simulink model "filecuaho"  (R2016b)
settings: Solver=VariableStepAuto  StartTime=0.0  StopTime=10.0  RelTol=1e-3
undefined symbols (not defined in the file): KACC_ACCT_CLR_NIDL_INIT, KACC_ACCUT_STATE_A, KACC_ACCUT_STATE_B, KACC_ACCUT_SW, KACC_ACTQSW, KACC_CLD, KACC_CLD_REQ_HYS, KACC_CLD_REQ_SW, KACC_COLPD, KACC_COMP_INRT, KACC_COMPTYPE_FIXED, KACC_COMPTYPE_VAR, KACC_CTTM_ACE, KACC_CTTM_ACON, KACC_CTTM_CRK, KACC_CTTM_FAN, KACC_CTTM_GRD, KACC_CTTM_IRS, KACC_CTTM_NAC, KACC_DIFFEVATEMPMAX, KACC_DIFFEVATEMPMIN, KACC_EVAT_ELSE, KACC_EVAT_ELSE_SW, KACC_EVATMPCUT_SW, KACC_EVATUPL_ELSE, KACC_EVATUPL_ELSE_SW, KACC_FANREQ_SW, KACC_FORCEDACON, KACC_HCAPS, KACC_HCAPS_HYS, KACC_HCCTTM, KACC_HCGRA, KACC_HCGRA_HYS, KACC_HCRGR, KACC_HCVS1, KACC_HCVS1_HYS, KACC_HCVS2, KACC_HCVS2_HYS, KACC_HEATUP_CE, KACC_HEATUP_CE_HYS, KACC_HEATUP_DRV2IDL, KACC_HEATUP_IDL2DRV, KACC_HEATUP_NE, KACC_HEATUP_NE_HYS, KACC_HIPS_ACOF, KACC_HIPS_ACON, KACC_LOPS_ACOF, KACC_LOPS_ACON, KACC_LYR3TR_ACHLD, KACC_NEW_RPM, KACC_OFDL_SW, KACC_OFDL_VCV, KACC_ONDL_SW, KACC_RECCP, KACC_RECCP_HYS, KACC_RECDLY, KACC_RECVS, KACC_S1_THWMAX, KACC_S1TM_THWULMT, KACC_SHLT_2CYL ... (+137)
libraries: lib2011b x727, SUBSYSTEM_LIB_CNV x30, SUBSYSTEM_LIB_ESC x2, SUBSYSTEM_LIB_AUX x1
(part 4 of 5)

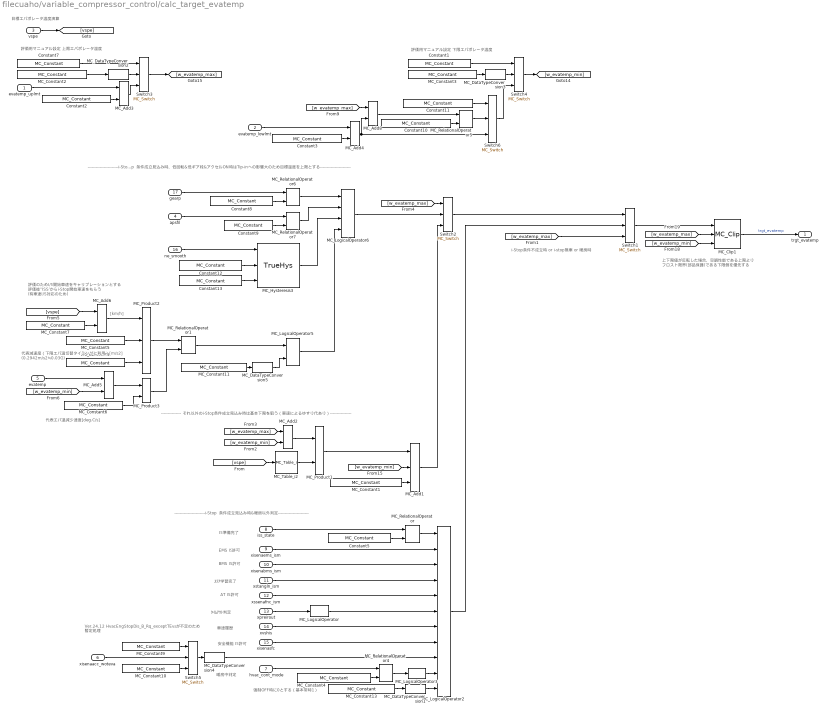
== system filecuaho/variable_compressor_control/calc_target_evatemp ==
  note: 評価用マニュアル設定 上限エバポレータ温度
  note: 評価用マニュアル設定 下限エバポレータ温度
  note: 上下限値が反転した場合、空調性能である上限より
      | フロスト限界(部品保護)である下限側を優先する
  note: 目標エバポレータ温度演算
  note: i-Stop条件不成立時 or i-stop無車 or 暖房時
  note: ---------------それ以外のi-Stop条件成立見込み時は基本下限を狙う（車速によるゆすり代あり）----------------
  note: -----------------------i-Stop条件成立見込み時、低回転&低ギア段&アクセルON時はTip-inへの影響大のため目標温度を上限とする-----------------------
  note: 代表減速度（下限エバ温切替タイミングに利用）[m/s2]
      | (0.2942m/s2≒0.03G)
  note: 代表エバ温減少速度[deg.C/s]
  note: 評価のためI/S開始車速をキャリブレーションとする
      | 評価後"ISS"からi-Stop開始車速をもらう
      | (有車速I/S対応のため)
  note: [km/h]
  note: Ver.24.12
      | HvacEngStopDis_B_Rq_exceptTEvaが不定のため
      | 暫定処理
  note: EMS IS許可
  note: BMS IS許可
  note: ｽﾃｱ学習完了
  note: AT IS許可
  note: ﾀｲﾑｱｳﾄ判定
  note: 車速履歴
  note: 安全機能 IS許可
  note: IS準備完了
  note: -----------------------i-Stop条件成立見込み時&暖房以外判定-----------------------
  note: 暖房中判定
  note: 強制OFF時に0とする（基本常時1）
  evatemp_uplmt : Inport
  evatemp_lowlmt : Inport  Port=2
  vspe : Inport  Port=3
  apsfil : Inport  Port=4
  evatemp : Inport  Port=5
  xisenaacc_woteva : Inport  Port=6
  hvac_cont_mode : Inport  Port=7
  iss_state : Inport  Port=8
  xisenaems_ism : Inport  Port=9
  xisenabms_ism : Inport  Port=10
  xstangln_ism : Inport  Port=11
  xssenafnc_ism : Inport  Port=12
  xpreirout : Inport  Port=13
  xvshis : Inport  Port=14
  xisenasfc : Inport  Port=15
  ne_smooth : Inport  Port=16
  gearp : Inport  Port=17
  Constant1 : lib2011b/Simulink Original/Sources/MC_Constant  Value=KACC_VCD_ETLO_MN  datatype=Inherit: Inherit from 'Constant value'  SampleTime=inf  FramePeriod=inf  OutMin=[]  OutMax=[]  OutDataTypeStr=Inherit: Inherit from 'Constant value'
  Constant10 : lib2011b/Simulink Original/Sources/MC_Constant  Value=KACC_VCD_EVA_DIFTEMP  datatype=Inherit: Inherit from 'Constant value'  SampleTime=inf  FramePeriod=inf  OutMin=[]  OutMax=[]  OutDataTypeStr=Inherit: Inherit from 'Constant value'
  Constant11 : lib2011b/Simulink Original/Sources/MC_Constant  Value=KACC_VCD_ETLO_TEMP  datatype=Inherit: Inherit from 'Constant value'  SampleTime=inf  FramePeriod=inf  OutMin=[]  OutMax=[]  OutDataTypeStr=Inherit: Inherit from 'Constant value'
  Constant12 : lib2011b/Simulink Original/Sources/MC_Constant  Value=KACC_VCD_NE  datatype=Inherit: Inherit from 'Constant value'  SampleTime=inf  FramePeriod=inf  OutMin=[]  OutMax=[]  OutDataTypeStr=Inherit: Inherit from 'Constant value'
  Constant13 : lib2011b/Simulink Original/Sources/MC_Constant  Value=KACC_VCD_NE_HYS  datatype=Inherit: Inherit from 'Constant value'  SampleTime=inf  FramePeriod=inf  OutMin=[]  OutMax=[]  OutDataTypeStr=Inherit: Inherit from 'Constant value'
  Constant2 : lib2011b/Simulink Original/Sources/MC_Constant  Value=KACC_VCD_ETHI_OFST  datatype=Inherit: Inherit from 'Constant value'  SampleTime=inf  FramePeriod=inf  OutMin=[]  OutMax=[]  OutDataTypeStr=Inherit: Inherit from 'Constant value'
  Constant3 : lib2011b/Simulink Original/Sources/MC_Constant  Value=KACC_VCD_ETLO_OFST  datatype=Inherit: Inherit from 'Constant value'  SampleTime=inf  FramePeriod=inf  OutMin=[]  OutMax=[]  OutDataTypeStr=Inherit: Inherit from 'Constant value'
  Constant5 : lib2011b/Simulink Original/Sources/MC_Constant  Value=KACC_VCD_ISNOTRDY  datatype=Inherit: Inherit from 'Constant value'  SampleTime=inf  FramePeriod=inf  OutMin=[]  OutMax=[]  OutDataTypeStr=Inherit: Inherit from 'Constant value'
  Constant7 : lib2011b/Simulink Original/Sources/MC_Constant  Value=KACC_VCD_ETHI_MN  datatype=Inherit: Inherit from 'Constant value'  SampleTime=inf  FramePeriod=inf  OutMin=[]  OutMax=[]  OutDataTypeStr=Inherit: Inherit from 'Constant value'
  Constant8 : lib2011b/Simulink Original/Sources/MC_Constant  Value=KACC_VCD_GEARP  datatype=Inherit: Inherit from 'Constant value'  SampleTime=inf  FramePeriod=inf  OutMin=[]  OutMax=[]  OutDataTypeStr=Inherit: Inherit from 'Constant value'
  Constant9 : lib2011b/Simulink Original/Sources/MC_Constant  Value=KACC_VCD_APS  datatype=Inherit: Inherit from 'Constant value'  SampleTime=inf  FramePeriod=inf  OutMin=[]  OutMax=[]  OutDataTypeStr=Inherit: Inherit from 'Constant value'
  MC_Add1 : lib2011b/Simulink Original/Math Operations/MC_Add  Inputs=+++  CollapseDim=1  SampleTime=-1  InputSameDT=on  OutMin=[]  OutMax=[]  OutDataTypeStr=single
  MC_Add{2,5..6,8} (4 alike) : lib2011b/Simulink Original/Math Operations/MC_Add  Inputs=+-  CollapseDim=1  SampleTime=-1  InputSameDT=on  OutMin=[]  OutMax=[]  OutDataTypeStr=single
  MC_Add3 : lib2011b/Simulink Original/Math Operations/MC_Add  Inputs=++  CollapseDim=1  SampleTime=-1  InputSameDT=on  OutMin=[]  OutMax=[]  OutDataTypeStr=single
  MC_Add4 : lib2011b/Simulink Original/Math Operations/MC_Add  Inputs=++  CollapseDim=1  SampleTime=-1  InputSameDT=on  OutMin=[]  OutMax=[]  OutDataTypeStr=single
  MC_Clip1 : lib2011b/Mazda Library/Other/MC_Clip
  MC_Constant1 : lib2011b/Simulink Original/Sources/MC_Constant  Value=KACC_VCD_TET_OFFSET  datatype=Inherit: Inherit from 'Constant value'  SampleTime=inf  FramePeriod=inf  OutMin=[]  OutMax=[]  OutDataTypeStr=Inherit: Inherit from 'Constant value'
  MC_Constant10 : lib2011b/Simulink Original/Sources/MC_Constant  Value=KACC_VCD_ISOFF  datatype=Inherit: Inherit from 'Constant value'  SampleTime=inf  FramePeriod=inf  OutMin=[]  OutMax=[]  OutDataTypeStr=Inherit: Inherit from 'Constant value'
  MC_Constant11 : lib2011b/Simulink Original/Sources/MC_Constant  Value=KACC_VCD_EVASP_SW  datatype=Inherit: Inherit from 'Constant value'  SampleTime=inf  FramePeriod=inf  OutMin=[]  OutMax=[]  OutDataTypeStr=Inherit: Inherit from 'Constant value'
  MC_Constant13 : lib2011b/Simulink Original/Sources/MC_Constant  Value=KACC_VCD_FORCEDOFF  datatype=Inherit: Inherit from 'Constant value'  SampleTime=inf  FramePeriod=inf  OutMin=[]  OutMax=[]  OutDataTypeStr=Inherit: Inherit from 'Constant value'
  MC_Constant2 : lib2011b/Simulink Original/Sources/MC_Constant  Value=KACC_VCD_ETHI_MNSW  datatype=Inherit: Inherit from 'Constant value'  SampleTime=inf  FramePeriod=inf  OutMin=[]  OutMax=[]  OutDataTypeStr=Inherit: Inherit from 'Constant value'
  MC_Constant3 : lib2011b/Simulink Original/Sources/MC_Constant  Value=KACC_VCD_ETLO_MNSW  datatype=Inherit: Inherit from 'Constant value'  SampleTime=inf  FramePeriod=inf  OutMin=[]  OutMax=[]  OutDataTypeStr=Inherit: Inherit from 'Constant value'
  MC_Constant4 : lib2011b/Simulink Original/Sources/MC_Constant  Value=KACC_VCD_HEATSTATE2  datatype=Inherit: Inherit from 'Constant value'  SampleTime=inf  FramePeriod=inf  OutMin=[]  OutMax=[]  OutDataTypeStr=Inherit: Inherit from 'Constant value'
  MC_Constant5 : lib2011b/Simulink Original/Sources/MC_Constant  Value=KACC_VCD_DISACC  datatype=Inherit: Inherit from 'Constant value'  SampleTime=inf  FramePeriod=inf  OutMin=[]  OutMax=[]  OutDataTypeStr=Inherit: Inherit from 'Constant value'
  MC_Constant6 : lib2011b/Simulink Original/Sources/MC_Constant  Value=KACC_VCD_DISET  datatype=Inherit: Inherit from 'Constant value'  SampleTime=inf  FramePeriod=inf  OutMin=[]  OutMax=[]  OutDataTypeStr=Inherit: Inherit from 'Constant value'
  MC_Constant7 : lib2011b/Simulink Original/Sources/MC_Constant  Value=KACC_VCD_ISSPD  datatype=Inherit: Inherit from 'Constant value'  SampleTime=inf  FramePeriod=inf  OutMin=[]  OutMax=[]  OutDataTypeStr=Inherit: Inherit from 'Constant value'
  MC_Constant8 : lib2011b/Simulink Original/Sources/MC_Constant  Value=3.6  datatype=single  SampleTime=inf  FramePeriod=inf  OutMin=[]  OutMax=[]  OutDataTypeStr=single
  MC_Constant9 : lib2011b/Simulink Original/Sources/MC_Constant  Value=KACC_VCD_ISON  datatype=Inherit: Inherit from 'Constant value'  SampleTime=inf  FramePeriod=inf  OutMin=[]  OutMax=[]  OutDataTypeStr=Inherit: Inherit from 'Constant value'
  MC_DataTypeConversion{1..5} (5 alike) : lib2011b/Simulink Original/Signal Attributes/MC_DataTypeConversion  OutMin=[]  OutMax=[]  OutDataTypeStr=boolean  Signaltype=boolean  ConvertRealWorld=Real World Value (RWV)  RndMeth=Zero  SampleTime=-1
  MC_Hysteresis3 : SUBSYSTEM_LIB_CNV/TrueHys
      settings: AttributesFormatString=True
  MC_LogicalOperator : lib2011b/Simulink Original/Logic and Bit Operations/MC_LogicalOperator  SelectedOperator=NOT  Inputs=2  SampleTime=-1  AllPortsSameDT=off  OutDataTypeStr=boolean
  MC_LogicalOperator2 : lib2011b/Simulink Original/Logic and Bit Operations/MC_LogicalOperator  SelectedOperator=AND  Inputs=11  SampleTime=-1  AllPortsSameDT=off  OutDataTypeStr=boolean
  MC_LogicalOperator3 : lib2011b/Simulink Original/Logic and Bit Operations/MC_LogicalOperator  SelectedOperator=NOT  Inputs=2  SampleTime=-1  AllPortsSameDT=off  OutDataTypeStr=boolean
  MC_LogicalOperator5 : lib2011b/Simulink Original/Logic and Bit Operations/MC_LogicalOperator  SelectedOperator=OR  Inputs=2  SampleTime=-1  AllPortsSameDT=off  OutDataTypeStr=boolean
  MC_LogicalOperator6 : lib2011b/Simulink Original/Logic and Bit Operations/MC_LogicalOperator  SelectedOperator=AND  Inputs=4  SampleTime=-1  AllPortsSameDT=off  OutDataTypeStr=boolean
  MC_Product1 : lib2011b/Simulink Original/Math Operations/MC_Product  Inputs=**  Multiplication=Element-wise(.*)  CollapseDim=1  SampleTime=-1  InputSameDT=on  OutMin=[]  OutMax=[]  OutDataTypeStr=single  RndMeth=Zero
  MC_Product2 : lib2011b/Simulink Original/Math Operations/MC_Product  Inputs=*//  Multiplication=Element-wise(.*)  CollapseDim=1  SampleTime=-1  InputSameDT=on  OutMin=[]  OutMax=[]  OutDataTypeStr=single  RndMeth=Zero
  MC_Product3 : lib2011b/Simulink Original/Math Operations/MC_Product  Inputs=*/  Multiplication=Element-wise(.*)  CollapseDim=1  SampleTime=-1  InputSameDT=on  OutMin=[]  OutMax=[]  OutDataTypeStr=single  RndMeth=Zero
  MC_RelationalOperator : lib2011b/Simulink Original/Logic and Bit Operations/MC_RelationalOperator  Operator=~=  SampleTime=-1  InputSameDT=on  OutDataTypeStr=boolean
  MC_RelationalOperator1 : lib2011b/Simulink Original/Logic and Bit Operations/MC_RelationalOperator  Operator=>  SampleTime=-1  InputSameDT=on  OutDataTypeStr=boolean
  MC_RelationalOperator4 : lib2011b/Simulink Original/Logic and Bit Operations/MC_RelationalOperator  Operator===  SampleTime=-1  InputSameDT=on  OutDataTypeStr=boolean
  MC_RelationalOperator5 : lib2011b/Simulink Original/Logic and Bit Operations/MC_RelationalOperator  Operator=>=  SampleTime=-1  InputSameDT=on  OutDataTypeStr=boolean
  MC_RelationalOperator6 : lib2011b/Simulink Original/Logic and Bit Operations/MC_RelationalOperator  Operator=>=  SampleTime=-1  InputSameDT=on  OutDataTypeStr=boolean
  MC_RelationalOperator7 : lib2011b/Simulink Original/Logic and Bit Operations/MC_RelationalOperator  Operator=>  SampleTime=-1  InputSameDT=on  OutDataTypeStr=boolean
  MC_Table_i2 : lib2011b/Simulink Original/Lookup Tables/MC_Table_i  Label=TACC_VCD_TTEMP_VSP  InputValues=TACC_VCD_TTEMP_VSP_X  calsw_x=on  OutputValues=TACC_VCD_TTEMP_VSP_Y  LsbValue=LSB_TACC_VCD_TTEMP_VSP_Y  OffsetValue=OFFSET_TACC_VCD_TTEMP_VSP_Y
      settings: AttributesFormatString=%<Label>\nX-axis %<calsw_x>
  Switch{1..6} (6 alike) : lib2011b/Simulink Original/Signal Routing/MC_Switch  Criteria=u2 ~= 0  Threshold=0  SampleTime=-1  InputSameDT=on  OutMin=[]  OutMax=[]  AllowDiffInputSizes=off
  trgt_evatemp : Outport
  wires:
  [vspe] -> MC_Table_i2/1
  MC_Product1/1 -> MC_Add1/1
  MC_Constant1/1 -> MC_Add1/3
  MC_Add2/1 -> MC_Product1/1
  MC_Table_i2/1 -> MC_Product1/2
  MC_DataTypeConversion2/1 -> Switch3/2
  MC_Constant2/1 -> MC_DataTypeConversion2/1
  Constant7/1 -> Switch3/1
  MC_DataTypeConversion3/1 -> Switch4/2
  MC_Constant3/1 -> MC_DataTypeConversion3/1
  Constant1/1 -> Switch4/1
  Switch3/1 -> [w_evatemp_max]
  [w_evatemp_max] -> MC_Clip1/2
  [w_evatemp_min] -> MC_Clip1/3
  [w_evatemp_min] -> MC_Add1/2
  MC_Clip1/1 -> trgt_evatemp/1  "trgt_evatemp"
  Switch1/1 -> MC_Clip1/1
  [w_evatemp_max] -> MC_Add2/1
  [w_evatemp_min] -> MC_Add2/2
  Constant2/1 -> MC_Add3/2
  MC_Add3/1 -> Switch3/3
  Constant3/1 -> MC_Add4/2
  evatemp_lowlmt/1 -> MC_Add4/1
  vspe/1 -> [vspe]
  MC_Constant5/1 -> MC_Product2/2
  MC_Product2/1 -> MC_RelationalOperator1/1
  [w_evatemp_min] -> MC_Add5/2
  evatemp/1 -> MC_Add5/1
  MC_Constant6/1 -> MC_Product3/2
  MC_Product3/1 -> MC_RelationalOperator1/2
  MC_Add5/1 -> MC_Product3/1
  MC_Constant7/1 -> MC_Add6/2
  MC_Add6/1 -> MC_Product2/1
  [vspe] -> MC_Add6/1
  MC_Constant8/1 -> MC_Product2/3
  iss_state/1 -> MC_RelationalOperator/1
  Constant5/1 -> MC_RelationalOperator/2
  xpreirout/1 -> MC_LogicalOperator/1
  MC_Constant9/1 -> Switch5/1
  MC_Constant10/1 -> Switch5/3
  xisenaacc_woteva/1 -> Switch5/2
  Switch5/1 -> MC_DataTypeConversion4/1
  hvac_cont_mode/1 -> MC_RelationalOperator4/1
  MC_Constant4/1 -> MC_RelationalOperator4/2
  MC_Constant13/1 -> MC_DataTypeConversion1/1
  MC_RelationalOperator4/1 -> MC_LogicalOperator3/1
  MC_RelationalOperator/1 -> MC_LogicalOperator2/1
  xisenaems_ism/1 -> MC_LogicalOperator2/2
  xisenabms_ism/1 -> MC_LogicalOperator2/3
  xstangln_ism/1 -> MC_LogicalOperator2/4
  xssenafnc_ism/1 -> MC_LogicalOperator2/5
  MC_LogicalOperator/1 -> MC_LogicalOperator2/6
  xvshis/1 -> MC_LogicalOperator2/7
  xisenasfc/1 -> MC_LogicalOperator2/8
  MC_DataTypeConversion4/1 -> MC_LogicalOperator2/9
  MC_LogicalOperator3/1 -> MC_LogicalOperator2/10
  MC_DataTypeConversion1/1 -> MC_LogicalOperator2/11
  Switch2/1 -> Switch1/1
  MC_LogicalOperator2/1 -> Switch1/2
  [w_evatemp_max] -> Switch1/3
  MC_Constant11/1 -> MC_DataTypeConversion5/1
  MC_RelationalOperator1/1 -> MC_LogicalOperator5/1
  MC_DataTypeConversion5/1 -> MC_LogicalOperator5/2
  evatemp_uplmt/1 -> MC_Add3/1
  [w_evatemp_max] -> MC_Add8/1
  MC_Add8/1 -> MC_RelationalOperator5/1
  Constant10/1 -> MC_RelationalOperator5/2
  MC_Add4/1 -> MC_Add8/2, Switch6/3
  Constant11/1 -> Switch6/1
  MC_RelationalOperator5/1 -> Switch6/2
  Switch6/1 -> Switch4/3
  Switch4/1 -> [w_evatemp_min]
  gearp/1 -> MC_RelationalOperator6/1
  Constant8/1 -> MC_RelationalOperator6/2
  Constant9/1 -> MC_RelationalOperator7/2
  MC_RelationalOperator6/1 -> MC_LogicalOperator6/1
  MC_RelationalOperator7/1 -> MC_LogicalOperator6/2
  MC_LogicalOperator5/1 -> MC_LogicalOperator6/4
  apsfil/1 -> MC_RelationalOperator7/1
  MC_LogicalOperator6/1 -> Switch2/2
  [w_evatemp_max] -> Switch2/1
  MC_Add1/1 -> Switch2/3
  ne_smooth/1 -> MC_Hysteresis3/1
  Constant12/1 -> MC_Hysteresis3/2
  Constant13/1 -> MC_Hysteresis3/3
  MC_Hysteresis3/1 -> MC_LogicalOperator6/3

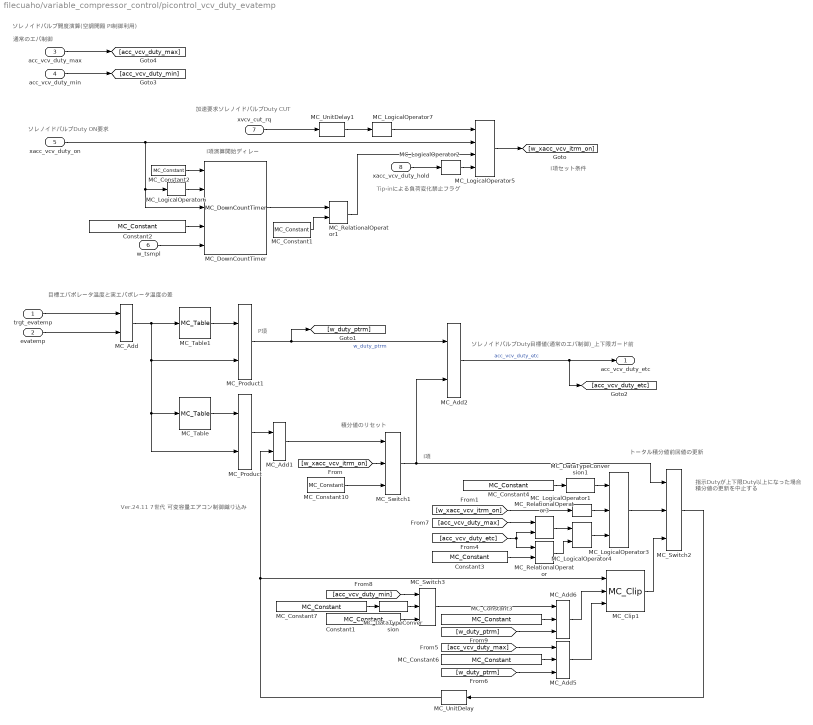
== system filecuaho/variable_compressor_control/picontrol_vcv_duty_evatemp ==
  note: 積分値のリセット
  note: 目標エバポレータ温度と実エバポレータ温度の差
  note: I項
  note: P項
  note: トータル積分値前回値の更新
  note: 通常のエバ制御
  note: ソレノイドバルブ開度演算(空調開殿 PI制御利用)
  note: 指示Dutyが上下限Duty以上になった場合
      | 積分値の更新を中止する
  note: ソレノイドバルブDuty目標値(通常のエバ制御)_上下限ガード前
  note: ソレノイドバルブDuty ON要求
  note: Ver.24.11
      | 7世代 可変容量エアコン制御織り込み
  note: I項セット条件
  note: I項演算開始ディレー
  note: 加速要求ソレノイドバルブDuty CUT
  note: Tip-inによる負荷変化禁止フラグ
  trgt_evatemp : Inport
  evatemp : Inport  Port=2
  acc_vcv_duty_max : Inport  Port=3
  acc_vcv_duty_min : Inport  Port=4
  xacc_vcv_duty_on : Inport  Port=5
  w_tsmpl : Inport  Port=6
  xvcv_cut_rq : Inport  Port=7
  xacc_vcv_duty_hold : Inport  Port=8
  Constant1 : lib2011b/Simulink Original/Sources/MC_Constant  Value=KACC_VCD_INIT  datatype=Inherit: Inherit from 'Constant value'  SampleTime=inf  FramePeriod=inf  OutMin=[]  OutMax=[]  OutDataTypeStr=Inherit: Inherit from 'Constant value'
  Constant2 : lib2011b/Simulink Original/Sources/MC_Constant  Value=KACC_VCD_ITSET_DLY  datatype=Inherit: Inherit from 'Constant value'  SampleTime=inf  FramePeriod=inf  OutMin=[]  OutMax=[]  OutDataTypeStr=Inherit: Inherit from 'Constant value'
  Constant3 : lib2011b/Simulink Original/Sources/MC_Constant  Value=KACC_VCD_INIT  datatype=Inherit: Inherit from 'Constant value'  SampleTime=inf  FramePeriod=inf  OutMin=[]  OutMax=[]  OutDataTypeStr=Inherit: Inherit from 'Constant value'
  MC_Add : lib2011b/Simulink Original/Math Operations/MC_Add  Inputs=+-  CollapseDim=1  SampleTime=-1  InputSameDT=on  OutMin=[]  OutMax=[]  OutDataTypeStr=single
  MC_Add1 : lib2011b/Simulink Original/Math Operations/MC_Add  Inputs=++  CollapseDim=1  SampleTime=-1  InputSameDT=on  OutMin=[]  OutMax=[]  OutDataTypeStr=single
  MC_Add2 : lib2011b/Simulink Original/Math Operations/MC_Add  Inputs=--  CollapseDim=1  SampleTime=-1  InputSameDT=on  OutMin=[]  OutMax=[]  OutDataTypeStr=single
  MC_Add5 : lib2011b/Simulink Original/Math Operations/MC_Add  Inputs=-+-  CollapseDim=1  SampleTime=-1  InputSameDT=on  OutMin=[]  OutMax=[]  OutDataTypeStr=single
  MC_Add6 : lib2011b/Simulink Original/Math Operations/MC_Add  Inputs=-+-  CollapseDim=1  SampleTime=-1  InputSameDT=on  OutMin=[]  OutMax=[]  OutDataTypeStr=single
  MC_Clip1 : lib2011b/Mazda Library/Other/MC_Clip
  MC_Constant1 : lib2011b/Simulink Original/Sources/MC_Constant  Value=0  datatype=single  SampleTime=inf  FramePeriod=inf  OutMin=[]  OutMax=[]  OutDataTypeStr=single
  MC_Constant10 : lib2011b/Simulink Original/Sources/MC_Constant  Value=0.0  datatype=single  SampleTime=inf  FramePeriod=inf  OutMin=[]  OutMax=[]  OutDataTypeStr=single
  MC_Constant2 : lib2011b/Simulink Original/Sources/MC_Constant  Value=false  datatype=Inherit: Inherit from 'Constant value'  SampleTime=inf  FramePeriod=inf  OutMin=[]  OutMax=[]  OutDataTypeStr=Inherit: Inherit from 'Constant value'
  MC_Constant3 : lib2011b/Simulink Original/Sources/MC_Constant  Value=KACC_VCD_ITMAX_OFST  datatype=Inherit: Inherit from 'Constant value'  SampleTime=inf  FramePeriod=inf  OutMin=[]  OutMax=[]  OutDataTypeStr=Inherit: Inherit from 'Constant value'
  MC_Constant4 : lib2011b/Simulink Original/Sources/MC_Constant  Value=KACC_VCD_ITUPD_SW  datatype=Inherit: Inherit from 'Constant value'  SampleTime=inf  FramePeriod=inf  OutMin=[]  OutMax=[]  OutDataTypeStr=Inherit: Inherit from 'Constant value'
  MC_Constant6 : lib2011b/Simulink Original/Sources/MC_Constant  Value=KACC_VCD_ITMIN_OFST  datatype=Inherit: Inherit from 'Constant value'  SampleTime=inf  FramePeriod=inf  OutMin=[]  OutMax=[]  OutDataTypeStr=Inherit: Inherit from 'Constant value'
  MC_Constant7 : lib2011b/Simulink Original/Sources/MC_Constant  Value=KACC_VCD_ITMAX_SW  datatype=Inherit: Inherit from 'Constant value'  SampleTime=inf  FramePeriod=inf  OutMin=[]  OutMax=[]  OutDataTypeStr=Inherit: Inherit from 'Constant value'
  MC_DataTypeConversion : lib2011b/Simulink Original/Signal Attributes/MC_DataTypeConversion  OutMin=[]  OutMax=[]  OutDataTypeStr=boolean  Signaltype=boolean  ConvertRealWorld=Real World Value (RWV)  RndMeth=Zero  SampleTime=-1
  MC_DataTypeConversion1 : lib2011b/Simulink Original/Signal Attributes/MC_DataTypeConversion  OutMin=[]  OutMax=[]  OutDataTypeStr=boolean  Signaltype=boolean  ConvertRealWorld=Real World Value (RWV)  RndMeth=Zero  SampleTime=-1
  MC_DownCountTimer : lib2011b/Mazda Library/Timer/MC_DownCountTimer
  MC_LogicalOperator{1..2,6..7} (4 alike) : lib2011b/Simulink Original/Logic and Bit Operations/MC_LogicalOperator  SelectedOperator=NOT  Inputs=2  SampleTime=-1  AllPortsSameDT=off  OutDataTypeStr=boolean
  MC_LogicalOperator3 : lib2011b/Simulink Original/Logic and Bit Operations/MC_LogicalOperator  SelectedOperator=OR  Inputs=3  SampleTime=-1  AllPortsSameDT=off  OutDataTypeStr=boolean
  MC_LogicalOperator4 : lib2011b/Simulink Original/Logic and Bit Operations/MC_LogicalOperator  SelectedOperator=AND  Inputs=2  SampleTime=-1  AllPortsSameDT=off  OutDataTypeStr=boolean
  MC_LogicalOperator5 : lib2011b/Simulink Original/Logic and Bit Operations/MC_LogicalOperator  SelectedOperator=AND  Inputs=4  SampleTime=-1  AllPortsSameDT=off  OutDataTypeStr=boolean
  MC_Product : lib2011b/Simulink Original/Math Operations/MC_Product  Inputs=**  Multiplication=Element-wise(.*)  CollapseDim=1  SampleTime=-1  InputSameDT=on  OutMin=[]  OutMax=[]  OutDataTypeStr=single  RndMeth=Zero
  MC_Product1 : lib2011b/Simulink Original/Math Operations/MC_Product  Inputs=**  Multiplication=Element-wise(.*)  CollapseDim=1  SampleTime=-1  InputSameDT=on  OutMin=[]  OutMax=[]  OutDataTypeStr=single  RndMeth=Zero
  MC_RelationalOperator : lib2011b/Simulink Original/Logic and Bit Operations/MC_RelationalOperator  Operator=>=  SampleTime=-1  InputSameDT=on  OutDataTypeStr=boolean
  MC_RelationalOperator1 : lib2011b/Simulink Original/Logic and Bit Operations/MC_RelationalOperator  Operator=<=  SampleTime=-1  InputSameDT=on  OutDataTypeStr=boolean
  MC_RelationalOperator3 : lib2011b/Simulink Original/Logic and Bit Operations/MC_RelationalOperator  Operator=>=  SampleTime=-1  InputSameDT=on  OutDataTypeStr=boolean
  MC_Switch1 : lib2011b/Simulink Original/Signal Routing/MC_Switch  Criteria=u2 ~= 0  Threshold=0  SampleTime=-1  InputSameDT=on  OutMin=[]  OutMax=[]  AllowDiffInputSizes=off
  MC_Switch2 : lib2011b/Simulink Original/Signal Routing/MC_Switch  Criteria=u2 ~= 0  Threshold=0  SampleTime=-1  InputSameDT=on  OutMin=[]  OutMax=[]  AllowDiffInputSizes=off
  MC_Switch3 : lib2011b/Simulink Original/Signal Routing/MC_Switch  Criteria=u2 ~= 0  Threshold=0  SampleTime=-1  InputSameDT=on  OutMin=[]  OutMax=[]  AllowDiffInputSizes=off
  MC_Table : lib2011b/Simulink Original/Lookup Tables/MC_Table  Label=TACC_VCD_ETC_KI  InputValues=TACC_VCD_ETC_KI_X  calsw_x=on  OutputValues=TACC_VCD_ETC_KI_Y
      settings: AttributesFormatString=%<Label>\nX-axis %<calsw_x>
  MC_Table1 : lib2011b/Simulink Original/Lookup Tables/MC_Table  Label=TACC_VCD_ETC_KP  InputValues=TACC_VCD_ETC_KP_X  calsw_x=on  OutputValues=TACC_VCD_ETC_KP_Y
      settings: AttributesFormatString=%<Label>\nX-axis %<calsw_x>
  MC_UnitDelay : lib2011b/Simulink Original/Discrete/MC_UnitDelay  InitialCondition=0  InputProcessing=Inherited  SampleTime=-1  StateName=delay_yclcn_b20m9502
      settings: StateMustResolveToSignalObject=off  StateStorageClass=ExportedGlobal
  MC_UnitDelay1 : lib2011b/Simulink Original/Discrete/MC_UnitDelay  InitialCondition=0  InputProcessing=Inherited  SampleTime=-1  StateName=delay_yclcn_b20m9503
      settings: StateMustResolveToSignalObject=off  StateStorageClass=ExportedGlobal
  acc_vcv_duty_etc : Outport
  wires:
  trgt_evatemp/1 -> MC_Add/1
  evatemp/1 -> MC_Add/2
  MC_Table/1 -> MC_Product/1
  MC_Product/1 -> MC_Add1/1
  MC_Table1/1 -> MC_Product1/1
  MC_Add/1 -> MC_Table1/1, MC_Product1/2, MC_Table/1, MC_Product/2
  MC_Product1/1 -> MC_Add2/1, [w_duty_ptrm]  "w_duty_ptrm"
  [w_xacc_vcv_itrm_on] -> MC_Switch1/2
  MC_Constant10/1 -> MC_Switch1/3
  MC_Add2/1 -> [acc_vcv_duty_etc], acc_vcv_duty_etc/1  "acc_vcv_duty_etc"
  MC_Switch1/1 -> MC_Switch2/1, MC_Add2/2
  MC_Clip1/1 -> MC_Switch2/3
  [acc_vcv_duty_etc] -> MC_RelationalOperator3/2, MC_RelationalOperator/1
  MC_UnitDelay/1 -> MC_Add1/2, MC_Clip1/1
  MC_Add1/1 -> MC_Switch1/1
  MC_Switch2/1 -> MC_UnitDelay/1
  acc_vcv_duty_max/1 -> [acc_vcv_duty_max]
  acc_vcv_duty_min/1 -> [acc_vcv_duty_min]
  [acc_vcv_duty_max] -> MC_RelationalOperator3/1
  Constant3/1 -> MC_RelationalOperator/2
  MC_RelationalOperator3/1 -> MC_LogicalOperator4/1
  MC_RelationalOperator/1 -> MC_LogicalOperator4/2
  MC_Constant4/1 -> MC_DataTypeConversion1/1
  MC_LogicalOperator3/1 -> MC_Switch2/2
  MC_LogicalOperator5/1 -> [w_xacc_vcv_itrm_on]
  MC_DataTypeConversion/1 -> MC_Switch3/2
  MC_Constant6/1 -> MC_Add5/2
  MC_Constant7/1 -> MC_DataTypeConversion/1
  [acc_vcv_duty_min] -> MC_Switch3/1
  [w_duty_ptrm] -> MC_Add5/3
  [acc_vcv_duty_max] -> MC_Add5/1
  MC_Switch3/1 -> MC_Add6/1
  MC_Constant3/1 -> MC_Add6/2
  [w_duty_ptrm] -> MC_Add6/3
  Constant1/1 -> MC_Switch3/3
  MC_Add6/1 -> MC_Clip1/2
  MC_Add5/1 -> MC_Clip1/3
  [w_xacc_vcv_itrm_on] -> MC_LogicalOperator1/1
  MC_DataTypeConversion1/1 -> MC_LogicalOperator3/1
  MC_LogicalOperator4/1 -> MC_LogicalOperator3/3
  MC_LogicalOperator1/1 -> MC_LogicalOperator3/2
  MC_Constant1/1 -> MC_RelationalOperator1/2
  MC_DownCountTimer/1 -> MC_RelationalOperator1/1
  MC_RelationalOperator1/1 -> MC_LogicalOperator5/3
  xacc_vcv_duty_on/1 -> MC_LogicalOperator6/1, MC_DownCountTimer/3, MC_LogicalOperator5/2
  MC_Constant2/1 -> MC_DownCountTimer/1
  MC_LogicalOperator6/1 -> MC_DownCountTimer/2
  w_tsmpl/1 -> MC_DownCountTimer/5
  Constant2/1 -> MC_DownCountTimer/4
  xvcv_cut_rq/1 -> MC_UnitDelay1/1
  MC_LogicalOperator7/1 -> MC_LogicalOperator5/1
  MC_UnitDelay1/1 -> MC_LogicalOperator7/1
  xacc_vcv_duty_hold/1 -> MC_LogicalOperator2/1
  MC_LogicalOperator2/1 -> MC_LogicalOperator5/4

== system filecuaho/variable_compressor_control/vcv_cut_req ==
  note: ●加速要求_容量Min制御
      | 以下の条件に当てはまった場合は可変容量エアコンの容量をMinとし、目標トルクを叶えることにより加速度の確保を狙う。
      | ・エンジン回転数（ne_smooth）＞1000rpm
      | ・最大エンジントルク（tqe_mx）-目標エンジントルク（des_tqei）＜20Nm
      | ・目標エンジントルク（des_tqei）＞70Nm
      | ・3≦ギア段（gearp）≦4
      | なお、AT変速中は無効化。
      | また、容量復帰時は一定の傾きを持たせる。
  note: vcvcut制御作動時間の算出
      | vcvcut制御作動中にエアコンカットが行われた際は、
      | エアコン復帰までの時間に対してvcvcut制御を行った時間分だけOffsetする
  note: vcvcut制御作動カウンタ
      | エアコンカット要求があった場合はリセット
  note: 加速要求込のDuty
  acc_vcv_duty_etc : Inport
  ne_smooth : Inport  Port=2
  tqe_mx : Inport  Port=3
  des_tqei : Inport  Port=4
  gearp : Inport  Port=5
  xsftflg : Inport  Port=6
  w_tsmpl : Inport  Port=7
  xaccuton : Inport  Port=8
  Constant1 : lib2011b/Simulink Original/Sources/MC_Constant  Value=KACC_VCD_INIT  datatype=Inherit: Inherit from 'Constant value'  SampleTime=inf  FramePeriod=inf  OutMin=[]  OutMax=[]  OutDataTypeStr=Inherit: Inherit from 'Constant value'
  MC_Constant5 : lib2011b/Simulink Original/Sources/MC_Constant  Value=KACC_VCVCUT_TIME  datatype=Inherit: Inherit from 'Constant value'  SampleTime=inf  FramePeriod=inf  OutMin=[]  OutMax=[]  OutDataTypeStr=Inherit: Inherit from 'Constant value'
  MC_Gain1 : lib2011b/Simulink Original/Math Operations/MC_Gain  Gain=1000  Multiplication=Element-wise(K.*u)  SampleTime=-1  OutMin=[]  OutMax=[]  ParamMin=[]  ParamMax=[]
  MC_LogicalOperator1 : lib2011b/Simulink Original/Logic and Bit Operations/MC_LogicalOperator  SelectedOperator=OR  Inputs=2  SampleTime=-1  AllPortsSameDT=off  OutDataTypeStr=boolean
  MC_LogicalOperator2 : lib2011b/Simulink Original/Logic and Bit Operations/MC_LogicalOperator  SelectedOperator=AND  Inputs=2  SampleTime=-1  AllPortsSameDT=off  OutDataTypeStr=boolean
  MC_LogicalOperator3 : lib2011b/Simulink Original/Logic and Bit Operations/MC_LogicalOperator  SelectedOperator=NOT  Inputs=2  SampleTime=-1  AllPortsSameDT=off  OutDataTypeStr=boolean
  MC_RelationalOperator1 : lib2011b/Simulink Original/Logic and Bit Operations/MC_RelationalOperator  Operator=<=  SampleTime=-1  InputSameDT=on  OutDataTypeStr=boolean
  MC_UpCountTimer : lib2011b/Mazda Library/Timer/MC_UpCountTimer  tmax=2147483647  tmax_bg=2147483647
      settings: AttributesFormatString=MAX = %<tmax>ms
  Switch3 : lib2011b/Simulink Original/Signal Routing/MC_Switch  Criteria=u2 ~= 0  Threshold=0  SampleTime=-1  InputSameDT=on  OutMin=[]  OutMax=[]  AllowDiffInputSizes=off
  vcvcut_req : Subsystem
  acc_vcv_duty_acl : Outport
  vcv_cut_time : Outport  Port=2
  xvcv_cut_rq : Outport  Port=3
  xvcv_cut_ini : Outport  Port=4
  wires:
  vcvcut_req/1(xvcv_cut_rq) -> [xvcv_cut_rq], MC_UpCountTimer/2, MC_LogicalOperator3/1
  w_tsmpl/1 -> [w_tsmpl]
  ne_smooth/1 -> vcvcut_req/1(ne_smooth)
  tqe_mx/1 -> vcvcut_req/2(tqe_mx)
  des_tqei/1 -> vcvcut_req/3(des_tqei)
  gearp/1 -> vcvcut_req/4(gearp)
  xsftflg/1 -> vcvcut_req/5(xsftflg)
  acc_vcv_duty_etc/1 -> [acc_vcv_duty_etc]
  xaccuton/1 -> [xaccuton]
  [acc_vcv_duty_acl] -> acc_vcv_duty_acl/1
  [vcv_cut_time] -> vcv_cut_time/1
  [xvcv_cut_rq] -> xvcv_cut_rq/1
  [w_tsmpl] -> MC_UpCountTimer/3
  MC_Constant5/1 -> MC_Gain1/1
  MC_UpCountTimer/1 -> MC_RelationalOperator1/1, [vcv_cut_time]  "vcv_cut_time"
  MC_Gain1/1 -> MC_RelationalOperator1/2
  Constant1/1 -> Switch3/1
  [acc_vcv_duty_etc] -> Switch3/3
  Switch3/1 -> [acc_vcv_duty_acl]  "acc_vcv_duty_acl"
  [xaccuton] -> MC_LogicalOperator1/1
  MC_LogicalOperator3/1 -> MC_LogicalOperator1/2
  MC_LogicalOperator1/1 -> MC_UpCountTimer/1
  MC_RelationalOperator1/1 -> MC_LogicalOperator2/1
  [xvcv_cut_rq] -> MC_LogicalOperator2/2
  MC_LogicalOperator2/1 -> Switch3/2, [xvcv_cut_ini]  "xvcv_cut_ini"
  [xvcv_cut_ini] -> xvcv_cut_ini/1

== system filecuaho/variable_compressor_control/vcv_duty_on_delay ==
  note: マグネットクラッチ締結前後のVCV Duty指示の切替は以下順番となる。
      | 　1.クラッチ締結後、"KACC_VCD_ONDLY"[ms]の遅れを持って、VCV Duty指示は"KACC_VCD_INIT"⇒acc_vcv_duty_minに切り替わる
      | 　2.VCV Duty指示出力後の次回演算(20ms)からは、VCV Duty指示はacc_vcv_duty_min⇒acc_vcv_duty_preに切り替わる
      | また、xcolc on→off時にはacc_vcv_dutyは強制的に初期値duty(KACC_VCD_INIT)となる
      | ※クラッチに対するOFFディレーについてはacc_xyclcn/set_init1内に設定
  note: Duty 目標値セットタイミング
  note: マグネットクラッチOFF⇒ON時VCV Duty目標値セットディレー
  note: ソレノイドバルブ 要求Duty ON状態
  xcolc : Inport
  xclcn : Inport  Port=2
  w_tsmpl : Inport  Port=3
  xaccuton : Inport  Port=4
  Constant12 : lib2011b/Simulink Original/Sources/MC_Constant  Value=false  datatype=Inherit: Inherit from 'Constant value'  SampleTime=inf  FramePeriod=inf  OutMin=[]  OutMax=[]  OutDataTypeStr=Inherit: Inherit from 'Constant value'
  Constant4 : lib2011b/Simulink Original/Sources/MC_Constant  Value=0  datatype=single  SampleTime=inf  FramePeriod=inf  OutMin=[]  OutMax=[]  OutDataTypeStr=single
  Constant5 : lib2011b/Simulink Original/Sources/MC_Constant  Value=KACC_VCD_ONDLY  datatype=Inherit: Inherit from 'Constant value'  SampleTime=inf  FramePeriod=inf  OutMin=[]  OutMax=[]  OutDataTypeStr=Inherit: Inherit from 'Constant value'
  DownTimer_cnt16 : lib2011b/Mazda Library/Timer/MC_DownCountTimer
      settings: AttributesFormatString=DownCountTimer
  MC_Edge : lib2011b/Mazda Library/Other/MC_Edge
  MC_LogicalOperator1 : lib2011b/Simulink Original/Logic and Bit Operations/MC_LogicalOperator  SelectedOperator=AND  Inputs=4  SampleTime=-1  AllPortsSameDT=off  OutDataTypeStr=boolean
  MC_LogicalOperator2 : lib2011b/Simulink Original/Logic and Bit Operations/MC_LogicalOperator  SelectedOperator=AND  Inputs=2  SampleTime=-1  AllPortsSameDT=off  OutDataTypeStr=boolean
  MC_LogicalOperator3 : lib2011b/Simulink Original/Logic and Bit Operations/MC_LogicalOperator  SelectedOperator=NOT  Inputs=2  SampleTime=-1  AllPortsSameDT=off  OutDataTypeStr=boolean
  MC_LogicalOperator5 : lib2011b/Simulink Original/Logic and Bit Operations/MC_LogicalOperator  SelectedOperator=NOT  Inputs=2  SampleTime=-1  AllPortsSameDT=off  OutDataTypeStr=boolean
  RelationalOperator13 : lib2011b/Simulink Original/Logic and Bit Operations/MC_RelationalOperator  Operator=<=  SampleTime=-1  InputSameDT=on  OutDataTypeStr=boolean
  xacc_vcv_duty_on : Outport
  wires:
  Constant12/1 -> DownTimer_cnt16/1
  [w_tsmpl] -> DownTimer_cnt16/5
  Constant4/1 -> RelationalOperator13/2
  DownTimer_cnt16/1 -> RelationalOperator13/1  "dutydl"
  Constant5/1 -> DownTimer_cnt16/4
  [xclcn] -> MC_LogicalOperator1/2
  [xcolc] -> MC_Edge/1
  [xcolc] -> MC_LogicalOperator1/1
  xclcn/1 -> [xclcn]
  w_tsmpl/1 -> [w_tsmpl]
  xcolc/1 -> [xcolc]
  MC_LogicalOperator1/1 -> xacc_vcv_duty_on/1  "xacc_vcv_duty_on"
  xaccuton/1 -> MC_LogicalOperator5/1
  [w_xaccuton_not] -> MC_LogicalOperator1/3
  RelationalOperator13/1 -> MC_LogicalOperator1/4
  MC_LogicalOperator5/1 -> [w_xaccuton_not]
  MC_Edge/1 -> MC_LogicalOperator2/1
  [xclcn] -> MC_LogicalOperator3/1
  MC_LogicalOperator3/1 -> MC_LogicalOperator2/2
  MC_LogicalOperator2/1 -> DownTimer_cnt16/2
  [xclcn] -> DownTimer_cnt16/3

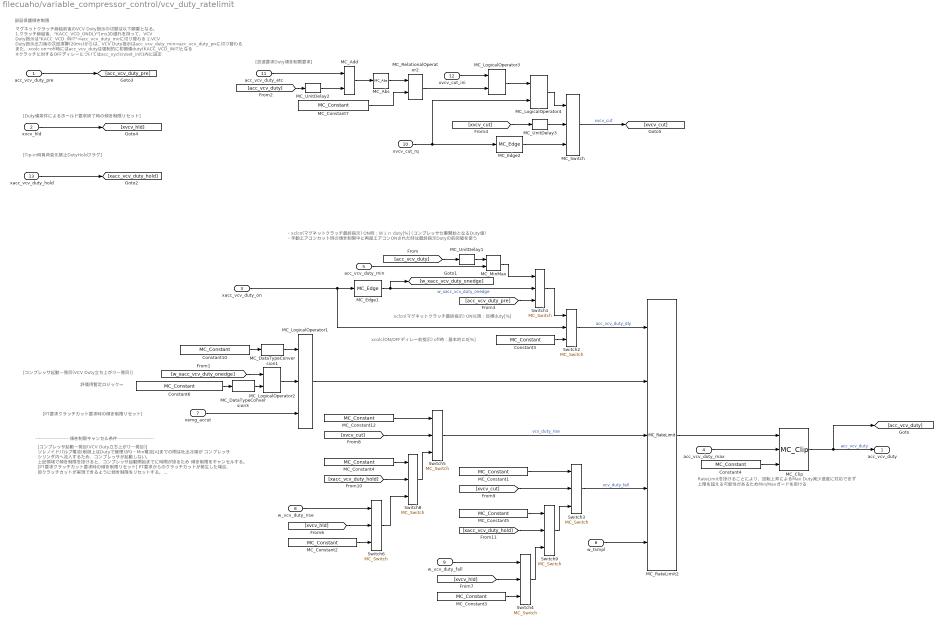
== system filecuaho/variable_compressor_control/vcv_duty_ratelimit ==
  note: 部品保護傾き制限
  note: ----------------------傾き制限キャンセル条件----------------------
  note: [コンプレッサ起動一発目(VCV Duty立ち上がり一発目)]
      | ソレノイドバルブ電流(制御上はDutyで管理)が0～Min電流[A]までの間は吐出冷媒が
      | コンプレッサ シリンダ内へ流入するため、コンプレッサが起動しない。
      | 上記領域で傾き制限を掛けると、コンプレッサ起動開始までに時間が掛るため
      | 傾き制限をキャンセルする。
      |
      | [PT要求クラッチカット要求時の傾き制限リセット]
      | PT要求からのクラッチカットが発生した場合、
      | 即クラッチカットが実現できるように傾き制限をリセットする。
      |
      | [Duty値条件によるホールド要求終了時の傾き制限リセット]
      | エアコン手動カット時にDutyがMin%以上であればステータスホールドを行うため傾き制限要。
      | この条件によるステータスホールドが完了（）すると傾き制限をリセットしDutyを瞬時に0%とする。
  note: [コンプレッサ起動一発目(VCV Duty立ち上がり一発目)]
  note: xcolc(ON/OFFディレー前指示) off時：基本的に0[%]
  note: xclcn(マグネットクラッチ最終指示) ON以降：目標duty[%]
  note: ・xclcn(マグネットクラッチ最終指示) ON時：Ｍｉｎ duty[%]
      | 　(コンプレッサ仕事開始となるDuty値)
      | ・手動エアコンカット時の傾き制限中に再度エアコンONされた時は最終指示Dutyの前回値を使う
  note: マグネットクラッチ締結前後のVCV Duty指示の切替は以下順番となる。
      | 　1.クラッチ締結後、"KACC_VCD_ONDLY"[ms]の遅れを持って、VCV Duty指示は"KACC_VCD_INIT"⇒acc_vcv_duty_minに切り替わる
      | 　2.VCV Duty指示出力後の次回演算(20ms)からは、VCV Duty指示はacc_vcv_duty_min⇒acc_vcv_duty_preに切り替わる
      | また、xcolc on→off時にはacc_vcv_dutyは強制的に初期値duty(KACC_VCD_INIT)となる
      | ※クラッチに対するOFFディレーについてはacc_xyclcn/set_init1内に設定
  note: RateLimitを掛けることにより、回転上昇によるMax Duty減少速度に対応できず
      | 上限を超える可能性があるためMin/Maxガードを掛ける
  note: 評価用暫定ロジック⇒
  note: [PT要求クラッチカット要求時の傾き制限リセット]
  note: [Duty値条件によるホールド要求終了時の傾き制限リセット]
  note: [加速要求Duty傾き制限要求]
  note: [Tip-in時負荷変化禁止DutyHoldフラグ]
  acc_vcv_duty_pre : Inport
  xvcv_hld : Inport  Port=2
  xacc_vcv_duty_on : Inport  Port=3
  acc_vcv_duty_max : Inport  Port=4
  acc_vcv_duty_min : Inport  Port=5
  w_tsmpl : Inport  Port=6
  xemg_accut : Inport  Port=7
  w_vcv_duty_rise : Inport  Port=8
  w_vcv_duty_fall : Inport  Port=9
  xvcv_cut_rq : Inport  Port=10
  acc_vcv_duty_etc : Inport  Port=11
  xvcv_cut_ini : Inport  Port=12
  xacc_vcv_duty_hold : Inport  Port=13
  Constant10 : lib2011b/Simulink Original/Sources/MC_Constant  Value=KACC_VCD_RLMT_SW  datatype=Inherit: Inherit from 'Constant value'  SampleTime=inf  FramePeriod=inf  OutMin=[]  OutMax=[]  OutDataTypeStr=Inherit: Inherit from 'Constant value'
  Constant3 : lib2011b/Simulink Original/Sources/MC_Constant  Value=KACC_VCD_INIT  datatype=Inherit: Inherit from 'Constant value'  SampleTime=inf  FramePeriod=inf  OutMin=[]  OutMax=[]  OutDataTypeStr=Inherit: Inherit from 'Constant value'
  Constant4 : lib2011b/Simulink Original/Sources/MC_Constant  Value=KACC_VCD_INIT  datatype=Inherit: Inherit from 'Constant value'  SampleTime=inf  FramePeriod=inf  OutMin=[]  OutMax=[]  OutDataTypeStr=Inherit: Inherit from 'Constant value'
  Constant6 : lib2011b/Simulink Original/Sources/MC_Constant  Value=KACC_VCD_RLMT_DUTY_SW1  datatype=Inherit: Inherit from 'Constant value'  SampleTime=inf  FramePeriod=inf  OutMin=[]  OutMax=[]  OutDataTypeStr=Inherit: Inherit from 'Constant value'
  MC_Abs : lib2011b/Simulink Original/Math Operations/MC_Abs  SampleTime=-1  OutMin=[]  OutMax=[]  OutDataTypeStr=single
  MC_Add : lib2011b/Simulink Original/Math Operations/MC_Add  Inputs=+-  CollapseDim=1  SampleTime=-1  InputSameDT=on  OutMin=[]  OutMax=[]  OutDataTypeStr=single
  MC_Clip : lib2011b/Mazda Library/Other/MC_Clip
  MC_Constant1 : lib2011b/Simulink Original/Sources/MC_Constant  Value=KACC_VCVCUT_FALL  datatype=Inherit: Inherit from 'Constant value'  SampleTime=inf  FramePeriod=inf  OutMin=[]  OutMax=[]  OutDataTypeStr=Inherit: Inherit from 'Constant value'
  MC_Constant12 : lib2011b/Simulink Original/Sources/MC_Constant  Value=KACC_VCVCUT_RISE  datatype=Inherit: Inherit from 'Constant value'  SampleTime=inf  FramePeriod=inf  OutMin=[]  OutMax=[]  OutDataTypeStr=Inherit: Inherit from 'Constant value'
  MC_Constant2 : lib2011b/Simulink Original/Sources/MC_Constant  Value=KACC_VCD_RISE  datatype=Inherit: Inherit from 'Constant value'  SampleTime=inf  FramePeriod=inf  OutMin=[]  OutMax=[]  OutDataTypeStr=Inherit: Inherit from 'Constant value'
  MC_Constant3 : lib2011b/Simulink Original/Sources/MC_Constant  Value=KACC_VCD_FALL  datatype=Inherit: Inherit from 'Constant value'  SampleTime=inf  FramePeriod=inf  OutMin=[]  OutMax=[]  OutDataTypeStr=Inherit: Inherit from 'Constant value'
  MC_Constant4 : lib2011b/Simulink Original/Sources/MC_Constant  Value=KACC_VCVHOLD_RISE  datatype=Inherit: Inherit from 'Constant value'  SampleTime=inf  FramePeriod=inf  OutMin=[]  OutMax=[]  OutDataTypeStr=Inherit: Inherit from 'Constant value'
  MC_Constant5 : lib2011b/Simulink Original/Sources/MC_Constant  Value=KACC_VCVHOLD_FALL  datatype=Inherit: Inherit from 'Constant value'  SampleTime=inf  FramePeriod=inf  OutMin=[]  OutMax=[]  OutDataTypeStr=Inherit: Inherit from 'Constant value'
  MC_Constant7 : lib2011b/Simulink Original/Sources/MC_Constant  Value=KACC_VCVCUT_DUTY  datatype=Inherit: Inherit from 'Constant value'  SampleTime=inf  FramePeriod=inf  OutMin=[]  OutMax=[]  OutDataTypeStr=Inherit: Inherit from 'Constant value'
  MC_DataTypeConversion1 : lib2011b/Simulink Original/Signal Attributes/MC_DataTypeConversion  OutMin=[]  OutMax=[]  OutDataTypeStr=boolean  Signaltype=boolean  ConvertRealWorld=Real World Value (RWV)  RndMeth=Zero  SampleTime=-1
  MC_DataTypeConversion3 : lib2011b/Simulink Original/Signal Attributes/MC_DataTypeConversion  OutMin=[]  OutMax=[]  OutDataTypeStr=boolean  Signaltype=boolean  ConvertRealWorld=Real World Value (RWV)  RndMeth=Zero  SampleTime=-1
  MC_Edge1 : lib2011b/Mazda Library/Other/MC_Edge
  MC_Edge2 : lib2011b/Mazda Library/Other/MC_Edge
  MC_LogicalOperator1 : lib2011b/Simulink Original/Logic and Bit Operations/MC_LogicalOperator  SelectedOperator=OR  Inputs=3  SampleTime=-1  AllPortsSameDT=off  OutDataTypeStr=boolean
  MC_LogicalOperator2 : lib2011b/Simulink Original/Logic and Bit Operations/MC_LogicalOperator  SelectedOperator=AND  Inputs=2  SampleTime=-1  AllPortsSameDT=off  OutDataTypeStr=boolean
  MC_LogicalOperator3 : lib2011b/Simulink Original/Logic and Bit Operations/MC_LogicalOperator  SelectedOperator=OR  Inputs=2  SampleTime=-1  AllPortsSameDT=off  OutDataTypeStr=boolean
  MC_LogicalOperator4 : lib2011b/Simulink Original/Logic and Bit Operations/MC_LogicalOperator  SelectedOperator=AND  Inputs=2  SampleTime=-1  AllPortsSameDT=off  OutDataTypeStr=boolean
  MC_MinMax : lib2011b/Simulink Original/Math Operations/MC_MinMax  Function=max  Inputs=2  SampleTime=-1  InputSameDT=on  OutMin=[]  OutMax=[]
  MC_RateLimit2 : lib2011b/Mazda Library/Other/MC_RateLimit
  MC_RelationalOperator2 : lib2011b/Simulink Original/Logic and Bit Operations/MC_RelationalOperator  Operator=>  SampleTime=-1  InputSameDT=on  OutDataTypeStr=boolean
  MC_Switch : lib2011b/Simulink Original/Signal Routing/MC_Switch  Criteria=u2 ~= 0  Threshold=0  SampleTime=-1  InputSameDT=on  OutMin=[]  OutMax=[]  AllowDiffInputSizes=off
  MC_UnitDelay1 : lib2011b/Simulink Original/Discrete/MC_UnitDelay  InitialCondition=0  InputProcessing=Inherited  SampleTime=-1  StateName=delay_yclcn_b20m9504
      settings: StateMustResolveToSignalObject=off  StateStorageClass=ExportedGlobal
  MC_UnitDelay2 : lib2011b/Simulink Original/Discrete/MC_UnitDelay  InitialCondition=0  InputProcessing=Inherited  SampleTime=-1  StateName=delay_yclcn_b20m9505
      settings: StateMustResolveToSignalObject=off  StateStorageClass=ExportedGlobal
  MC_UnitDelay3 : lib2011b/Simulink Original/Discrete/MC_UnitDelay  InitialCondition=0  InputProcessing=Inherited  SampleTime=-1  StateName=delay_yclcn_b20m9506
      settings: StateMustResolveToSignalObject=off  StateStorageClass=ExportedGlobal
  Switch{1..6,8..9} (8 alike) : lib2011b/Simulink Original/Signal Routing/MC_Switch  Criteria=u2 ~= 0  Threshold=0  SampleTime=-1  InputSameDT=on  OutMin=[]  OutMax=[]  AllowDiffInputSizes=off
  acc_vcv_duty : Outport
  wires:
  w_tsmpl/1 -> MC_RateLimit2/5
  Constant10/1 -> MC_DataTypeConversion1/1
  MC_RateLimit2/1 -> MC_Clip/1
  MC_DataTypeConversion1/1 -> MC_LogicalOperator1/1
  [w_xacc_vcv_duty_onedge] -> MC_LogicalOperator2/1
  MC_LogicalOperator2/1 -> MC_LogicalOperator1/2
  xacc_vcv_duty_on/1 -> MC_Edge1/1, Switch2/2
  Switch1/1 -> Switch2/1
  Switch2/1 -> MC_RateLimit2/1  "acc_vcv_duty_dly"
  MC_Edge1/1 -> Switch1/2, [w_xacc_vcv_duty_onedge]  "w_xacc_vcv_duty_onedge"
  [acc_vcv_duty_pre] -> Switch1/3
  acc_vcv_duty_max/1 -> MC_Clip/2
  Constant4/1 -> MC_Clip/3
  Constant6/1 -> MC_DataTypeConversion3/1
  MC_DataTypeConversion3/1 -> MC_LogicalOperator2/2
  MC_UnitDelay1/1 -> MC_MinMax/1
  [acc_vcv_duty] -> MC_UnitDelay1/1
  acc_vcv_duty_min/1 -> MC_MinMax/2
  MC_MinMax/1 -> Switch1/1
  Constant3/1 -> Switch2/3
  xemg_accut/1 -> MC_LogicalOperator1/3
  [acc_vcv_duty] -> MC_UnitDelay2/1
  acc_vcv_duty_pre/1 -> [acc_vcv_duty_pre]
  MC_Constant2/1 -> Switch6/3
  xvcv_hld/1 -> [xvcv_hld]
  MC_Constant3/1 -> Switch4/3
  MC_LogicalOperator1/1 -> MC_RateLimit2/2
  Switch5/1 -> MC_RateLimit2/3  "vcv_duty_rise"
  Switch3/1 -> MC_RateLimit2/4  "vcv_duty_fall"
  MC_Constant12/1 -> Switch5/1
  [xvcv_cut] -> Switch5/2
  w_vcv_duty_rise/1 -> Switch6/1
  [xvcv_hld] -> Switch6/2
  MC_Constant1/1 -> Switch3/1
  [xvcv_cut] -> Switch3/2
  w_vcv_duty_fall/1 -> Switch4/1
  [xvcv_hld] -> Switch4/2
  MC_Constant7/1 -> MC_RelationalOperator2/2
  MC_Add/1 -> MC_Abs/1
  MC_UnitDelay2/1 -> MC_Add/2
  MC_Abs/1 -> MC_RelationalOperator2/1
  MC_RelationalOperator2/1 -> MC_LogicalOperator3/2
  MC_Switch/1 -> [xvcv_cut]  "xvcv_cut"
  acc_vcv_duty_etc/1 -> MC_Add/1
  xvcv_cut_rq/1 -> MC_Edge2/1, MC_LogicalOperator4/2
  [xvcv_cut] -> MC_UnitDelay3/1
  MC_LogicalOperator3/1 -> MC_LogicalOperator4/1
  MC_LogicalOperator4/1 -> MC_Switch/1
  MC_UnitDelay3/1 -> MC_Switch/2
  xvcv_cut_ini/1 -> MC_LogicalOperator3/1
  MC_Edge2/1 -> MC_Switch/3
  xacc_vcv_duty_hold/1 -> [xacc_vcv_duty_hold]
  MC_Constant4/1 -> Switch8/1
  [xacc_vcv_duty_hold] -> Switch8/2
  Switch6/1 -> Switch8/3
  Switch8/1 -> Switch5/3
  MC_Constant5/1 -> Switch9/1
  [xacc_vcv_duty_hold] -> Switch9/2
  Switch4/1 -> Switch9/3
  Switch9/1 -> Switch3/3
  MC_Clip/1 -> acc_vcv_duty/1, [acc_vcv_duty]  "acc_vcv_duty"

== system filecuaho/acc_tqe/ac_inertia_torque/ac_torque_estimation_inrtia ==
  note: roll/min⇒rad/sec
  note: マグネットクラッチ締結時間[ms]
  note: 角加速度[rad/sec^2]
  note: msec⇒sec
  note: マグネットクラッチON時のイナーシャ
      | [kg・mm^2]
  note: kg・mm^2⇒kg・m^2
  note: イナーシャ[kg・m^2]
  note: マグネットクラッチOFF:0
      | マグネットクラッチ締結中(締結時間より): エアコン回転数(エンジン回転数×プーリー比)を保持
      | マグネットクラッチ締結完了:0
  nac : Inport
  xcolc : Inport  Port=2
  clacdl : Inport  Port=3
  w_tsmpl : Inport  Port=4
  Constant1 : lib2011b/Simulink Original/Sources/MC_Constant  Value=false  datatype=Inherit: Inherit from 'Constant value'  SampleTime=inf  FramePeriod=inf  OutMin=[]  OutMax=[]  OutDataTypeStr=Inherit: Inherit from 'Constant value'
  Constant2 : lib2011b/Simulink Original/Sources/MC_Constant  Value=0.1047  datatype=single  SampleTime=inf  FramePeriod=inf  OutMin=[]  OutMax=[]  OutDataTypeStr=single
  Constant3 : lib2011b/Simulink Original/Sources/MC_Constant  Value=1000.0  datatype=single  SampleTime=inf  FramePeriod=inf  OutMin=[]  OutMax=[]  OutDataTypeStr=single
  Constant4 : lib2011b/Simulink Original/Sources/MC_Constant  Value=1000000.0  datatype=single  SampleTime=inf  FramePeriod=inf  OutMin=[]  OutMax=[]  OutDataTypeStr=single
  Constant5 : lib2011b/Simulink Original/Sources/MC_Constant  Value=true  datatype=Inherit: Inherit from 'Constant value'  SampleTime=inf  FramePeriod=inf  OutMin=[]  OutMax=[]  OutDataTypeStr=Inherit: Inherit from 'Constant value'
  Constant6 : lib2011b/Simulink Original/Sources/MC_Constant  Value=0  datatype=single  SampleTime=inf  FramePeriod=inf  OutMin=[]  OutMax=[]  OutDataTypeStr=single
  Constant8 : lib2011b/Simulink Original/Sources/MC_Constant  Value=0  datatype=single  SampleTime=inf  FramePeriod=inf  OutMin=[]  OutMax=[]  OutDataTypeStr=single
  MC_Add : lib2011b/Simulink Original/Math Operations/MC_Add  Inputs=++  CollapseDim=1  SampleTime=-1  InputSameDT=on  OutMin=[]  OutMax=[]  OutDataTypeStr=single
  MC_Constant1 : lib2011b/Simulink Original/Sources/MC_Constant  Value=KACC_COMP_INRT  datatype=Inherit: Inherit from 'Constant value'  SampleTime=inf  FramePeriod=inf  OutMin=[]  OutMax=[]  OutDataTypeStr=Inherit: Inherit from 'Constant value'
  MC_DownCountTimer : lib2011b/Mazda Library/Timer/MC_DownCountTimer
  MC_Edge : lib2011b/Mazda Library/Other/MC_Edge
  MC_Product2 : lib2011b/Simulink Original/Math Operations/MC_Product  Inputs=**  Multiplication=Element-wise(.*)  CollapseDim=1  SampleTime=-1  OutMin=[]  OutMax=[]  OutDataTypeStr=single  RndMeth=Zero
  MC_Product3 : lib2011b/Simulink Original/Math Operations/MC_Product  Inputs=*/  Multiplication=Element-wise(.*)  CollapseDim=1  SampleTime=-1  OutMin=[]  OutMax=[]  OutDataTypeStr=single  RndMeth=Zero
  MC_Product4 : lib2011b/Simulink Original/Math Operations/MC_Product  Inputs=*/  Multiplication=Element-wise(.*)  CollapseDim=1  SampleTime=-1  OutMin=[]  OutMax=[]  OutDataTypeStr=single  RndMeth=Zero
  MC_Product5 : lib2011b/Simulink Original/Math Operations/MC_Product  Inputs=*/  Multiplication=Element-wise(.*)  CollapseDim=1  SampleTime=-1  OutMin=[]  OutMax=[]  OutDataTypeStr=single  RndMeth=Zero
  MC_Product6 : lib2011b/Simulink Original/Math Operations/MC_Product  Inputs=**  Multiplication=Element-wise(.*)  CollapseDim=1  SampleTime=-1  OutMin=[]  OutMax=[]  OutDataTypeStr=single  RndMeth=Zero
  MC_RelationalOperator : lib2011b/Simulink Original/Logic and Bit Operations/MC_RelationalOperator  Operator=>  SampleTime=-1  InputSameDT=on  OutDataTypeStr=boolean
  MC_Switch : lib2011b/Simulink Original/Signal Routing/MC_Switch  Criteria=u2 ~= 0  Threshold=0  SampleTime=-1  InputSameDT=on  OutMin=[]  OutMax=[]  AllowDiffInputSizes=off
  MC_Switch2 : lib2011b/Simulink Original/Signal Routing/MC_Switch  Criteria=u2 ~= 0  Threshold=0  SampleTime=-1  InputSameDT=on  OutMin=[]  OutMax=[]  AllowDiffInputSizes=off
  MC_Table_i : lib2011b/Simulink Original/Lookup Tables/MC_Table_i  Label=TACC_TIME_CLCN  InputValues=TACC_TIME_CLCN_X  calsw_x=on  OutputValues=TACC_TIME_CLCN_Y  LsbValue=LSB_TACC_TIME_CLCN_Y  OffsetValue=OFFSET_TACC_TIME_CLCN_Y
      settings: AttributesFormatString=%<Label>\nX-axis %<calsw_x>
  MC_UnitDelay : lib2011b/Simulink Original/Discrete/MC_UnitDelay  InitialCondition=0  InputProcessing=Inherited  SampleTime=-1  StateName=delay_yclcn_b20m9495
      settings: StateMustResolveToSignalObject=off  StateStorageClass=ExportedGlobal
  tqac_new_inrt : Outport
  wires:
  Constant2/1 -> MC_Product2/2
  MC_Product2/1 -> MC_Product3/1
  Constant3/1 -> MC_Product4/2
  MC_Product4/1 -> MC_Product3/2
  Constant4/1 -> MC_Product5/2
  MC_Constant1/1 -> MC_Product5/1
  MC_Product3/1 -> MC_Product6/2
  MC_Product5/1 -> MC_Product6/1
  MC_Product6/1 -> tqac_new_inrt/1  "tqac_new_inrt"
  MC_UnitDelay/1 -> MC_Switch/1
  MC_Switch/1 -> MC_UnitDelay/1, MC_Switch2/1
  MC_RelationalOperator/1 -> MC_Switch/2, MC_Switch2/2
  w_tsmpl/1 -> MC_DownCountTimer/5
  MC_Edge/1 -> MC_DownCountTimer/2
  [nac] -> MC_Table_i/1
  MC_DownCountTimer/1 -> MC_RelationalOperator/1
  Constant6/1 -> MC_RelationalOperator/2
  Constant5/1 -> MC_DownCountTimer/3
  [nac] -> MC_Switch/3
  nac/1 -> [nac]
  xcolc/1 -> [xcolc]
  Constant8/1 -> MC_Switch2/3
  MC_Switch2/1 -> MC_Product2/1
  MC_Table_i/1 -> MC_Product4/1, MC_Add/2
  MC_Add/1 -> MC_DownCountTimer/4
  clacdl/1 -> MC_Add/1
  Constant1/1 -> MC_DownCountTimer/1
  [xcolc] -> MC_Edge/1
